simulink model "SPGF_FSK_0000_R2022b"  (R2022b)
settings: Solver=ode4  StartTime=0.0  StopTime=1.4  FixedStep=50e-6/50  RelTol=1e-3  EnableMultiTasking=on
undefined symbols (not defined in the file): D11, Delta
libraries: spsSeriesRLCBranchLib x1646, spsGroundLib x360, spsStairGeneratorLib x147, spsIdealSwitchLib x145, spsCurrentMeasurementLib x145, spsUniversalBridgeLib x76, spsThreePhaseSeriesRLCLoadLib x57, simulink x45, spsBistableLib x36, spsSequenceAnalyzerLib x31, spsThreePhaseParallelRLCLoadLib x20, spsThreePhaseTransformerTwoWindingsLib x20
(part 28 of 40)

== system SPGF_FSK_0000_R2022b/W42/DPL ==
  Ccs2/1 : spsSeriesRLCBranchLib/Series RLC Branch  LConnTagsString=__new0  RConnTagsString=__new0  BranchType=R  Resistance=-Rg_matrix(3,4)*2  Inductance=1e-3  SetiL0=off  InitialCurrent=0  Capacitance=Rg_matrix(3,4)*2  Setx0=off  InitialVoltage=0  Measurements=None
  Ccs2/3 : spsSeriesRLCBranchLib/Series RLC Branch  LConnTagsString=__new0  RConnTagsString=__new0  BranchType=R  Resistance=-Rg_matrix(3,4)*2  Inductance=1e-3  SetiL0=off  InitialCurrent=0  Capacitance=Rg_matrix(3,4)*2  Setx0=off  InitialVoltage=0  Measurements=None
  Ccs3/1 : spsSeriesRLCBranchLib/Series RLC Branch  LConnTagsString=__new0  RConnTagsString=__new0  BranchType=R  Resistance=-Rg_matrix(5,6)*2  Inductance=1e-3  SetiL0=off  InitialCurrent=0  Capacitance=-C_matrix(5,6)/2  Setx0=off  InitialVoltage=0  Measurements=None
  Ccs3/3 : spsSeriesRLCBranchLib/Series RLC Branch  LConnTagsString=__new0  RConnTagsString=__new0  BranchType=R  Resistance=-Rg_matrix(5,6)*2  Inductance=1e-3  SetiL0=off  InitialCurrent=0  Capacitance=-C_matrix(5,6)/2  Setx0=off  InitialVoltage=0  Measurements=None
  DPL : spsDistributedParametersLineLib/Distributed Parameters Line  Phases=6  Length=LineLength  Frequency=Frequency  Resistance=R_matrix  Inductance=L_matrix  Capacitance=C_matrix  x1=[-1.8e-05 -1.53172591975226 5050.73263956514 0 -2664.13868695277 4776.09397012156 0;-1.75e-05 -1.53217240636053 5052.15465053998 0 -2664.88876317377 4775.67515317595 0;-1.7e-05 -1.53261885516397 5053.5765368579 0 -2665.63877364128 4775.25621839527 0;-1.65e-05 -1.53306526615155 5054.99829848381 0 -2666.38871833678 4774.83716578987 0;-1.6e-05 -1.53351163931226 5056.41993538264 0 -2667.13859724178 4774.41799537009 0;-1.55e-05 -1.53395797463509 5057.84144751931 0 -2667.88841033777 4773.99870714626 0;-1.5e-05 -1.53440427210902 5059.26283485875 0 -2668.63815760626 4773.57930112874 0;-1.45e-05 -1.53485053172304 5060.68409736588 0 -2669.38783902873 4773.15977732786 0;-1.4e-05 -1.53529675346615 5062.10523500563 0 -2670.13745458671 4772.74013575399 0;-1.35e-05 -1.53574293732732 5063.52624774295 0 -2670.88700426168 4772.32037641749 0;-1.3e-05 -1.53618908329556 5064.94713554276 0 -2671.63648803516 4771.90049932869 0;-1.25e-05 -1.53663519135985 5066.36789837001 0 -2672.38590588864 4771.48050449797 0;-1.2e-05 -1.53708126150919 5067.78853618965 0 -2673.13525780365 4771.06039193568 0;-1.15e-05 -1.53752729373257 5069.20904896661 0 -2673.8845437617 4770.6401616522 0;-1.1e-05 -1.53797328801899 5070.62943666586 0 -2674.63376374428 4770.2198136579 0;-1.05e-05 -1.53841924435743 5072.04969925233 0 -2675.38291773292 4769.79934796314 0;-1e-05 -1.5388651627369 5073.469836691 0 -2676.13200570914 4769.37876457829 0;-9.5e-06 -1.5393110431464 5074.88984894682 0 -2676.88102765444 4768.95806351374 0;-9e-06 -1.53975688557491 5076.30973598475 0 -2677.62998355035 4768.53724477987 0;-8.5e-06 -1.54020269001145 5077.72949776976 0 -2678.37887337839 4768.11630838706 0;-8e-06 -1.54064845644501 5079.14913426682 0 -2679.12769712009 4767.69525434569 0;-7.5e-06 -1.5410941848646 5080.56864544089 0 -2679.87645475695 4767.27408266616 0;-7e-06 -1.54153987525921 5081.98803125696 0 -2680.62514627051 4766.85279335886 0;-6.5e-06 -1.54198552761784 5083.40729168 0 -2681.3737716423 4766.43138643418 0;-6e-06 -1.54243114192951 5084.82642667499 0 -2682.12233085385 4766.00986190251 0;-5.5e-06 -1.54287671818322 5086.24543620692 0 -2682.87082388668 4765.58821977427 0;-5e-06 -1.54332225636797 5087.66432024077 0 -2683.61925072232 4765.16646005985 0;-4.5e-06 -1.54376775647277 5089.08307874154 0 -2684.36761134231 4764.74458276967 0;-4e-06 -1.54421321848662 5090.50171167422 -12.0892925887177 -2685.11590572819 4764.32258791412 0;-3.5e-06 -1.54465864239855 5091.9202190038 -12.0928204348561 -2685.86413386149 4763.90047550362 0;-3e-06 -1.54510402819755 5093.33860069529 -12.0963479826162 -2686.61229572375 4763.4782455486 0;-2.5e-06 -1.54554937587263 5094.75685671368 -12.0998752319109 -2687.3603912965 4763.05589805946 -9026.79288136857;-2e-06 -1.54599468541281 5096.17498702399 -12.1034021826531 -2688.1084205613 4762.63343304662 -9025.99223903892;-1.5e-06 -1.54643995680711 5097.59299159122 -12.1069288347558 -2688.85638349968 4762.21085052052 -9025.19137400184;-1e-06 -1.54688519004452 5099.01087038039 -12.110455188132 -2689.60428009319 4761.78815049157 -9024.39028627708;-5e-07 -1.54733038511408 5100.4286233565 -12.1139812426947 -2690.35211032337 4761.36533297021 -9023.58897588442]  x2=[-1.8e-05 -1.53125275621797 5053.5845076313 0 -2665.64297802649 4783.13395193963 0;-1.75e-05 -1.53170105381603 5055.00866650009 0 -2666.39418720933 4782.71500217531 0;-1.7e-05 -1.53214931362089 5056.43270064153 0 -2667.14533060154 4782.29593440223 0;-1.65e-05 -1.53259753562148 5057.8566100205 0 -2667.89640818457 4781.87674863072 0;-1.6e-05 -1.53304571980674 5059.28039460186 0 -2668.6474199399 4781.45744487113 0;-1.55e-05 -1.53349386616561 5060.70405435048 0 -2669.39836584899 4781.03802313381 0;-1.5e-05 -1.53394197468704 5062.12758923123 0 -2670.14924589332 4780.61848342911 0;-1.45e-05 -1.53439004535997 5063.55099920899 0 -2670.90006005435 4780.19882576737 0;-1.4e-05 -1.53483807817334 5064.97428424864 0 -2671.65080831357 4779.77905015896 0;-1.35e-05 -1.5352860731161 5066.39744431506 0 -2672.40149065245 4779.35915661423 0;-1.3e-05 -1.53573403017719 5067.82047937313 0 -2673.15210705246 4778.93914514353 0;-1.25e-05 -1.53618194934557 5069.24338938775 0 -2673.90265749509 4778.51901575724 0;-1.2e-05 -1.53662983061017 5070.66617432379 0 -2674.65314196181 4778.09876846572 0;-1.15e-05 -1.53707767395996 5072.08883414617 0 -2675.40356043412 4777.67840327933 0;-1.1e-05 -1.53752547938387 5073.51136881976 0 -2676.15391289349 4777.25792020846 0;-1.05e-05 -1.53797324687086 5074.93377830949 0 -2676.9041993214 4776.83731926347 0;-1e-05 -1.53842097640989 5076.35606258024 0 -2677.65441969936 4776.41660045475 0;-9.5e-06 -1.53886866798989 5077.77822159693 0 -2678.40457400884 4775.99576379267 0;-9e-06 -1.53931632159984 5079.20025532446 0 -2679.15466223133 4775.57480928762 0;-8.5e-06 -1.53976393722868 5080.62216372775 0 -2679.90468434834 4775.15373694998 0;-8e-06 -1.54021151486536 5082.04394677171 0 -2680.65464034134 4774.73254679015 0;-7.5e-06 -1.54065905449885 5083.46560442126 0 -2681.40453019185 4774.31123881852 0;-7e-06 -1.5411065561181 5084.88713664133 0 -2682.15435388134 4773.88981304547 0;-6.5e-06 -1.54155401971207 5086.30854339683 0 -2682.90411139134 4773.46826948142 0;-6e-06 -1.54200144526972 5087.72982465271 0 -2683.65380270333 4773.04660813676 0;-5.5e-06 -1.54244883278001 5089.15098037388 0 -2684.40342779881 4772.6248290219 0;-5e-06 -1.5428961822319 5090.57201052529 0 -2685.1529866593 4772.20293214723 0;-4.5e-06 -1.54334349361435 5091.99291507186 0 -2685.90247926629 4771.78091752318 0;-4e-06 -1.54379076691633 5093.41369397855 -12.0824675797471 -2686.65190560129 4771.35878516016 0;-3.5e-06 -1.5442380021268 5094.83434721029 -12.0860127319719 -2687.40126564582 4770.93653506858 0;-3e-06 -1.54468519923472 5096.25487473204 -12.0895575859862 -2688.15055938137 4770.51416725885 0;-2.5e-06 -1.54513235822907 5097.67527650873 -12.0931021417027 -2688.89978678947 4770.09168174141 -9040.12687605904;-2e-06 -1.5455794790988 5099.09555250533 -12.0966463990338 -2689.64894785163 4769.66907852667 -9039.32597181351;-1.5e-06 -1.54602656183288 5100.51570268679 -12.1001903578921 -2690.39804254936 4769.24635762507 -9038.52484453156;-1e-06 -1.54647360642029 5101.93572701807 -12.1037340181902 -2691.14707086418 4768.82351904703 -9037.72349423295;-5e-07 -1.54692061285 5103.35562546413 -12.1072773798407 -2691.89603277761 4768.40056280298 -9036.92192093744]  x3=[-1.8e-05 0.002122617198667 46.2927341881195 0 -221.66475085935 447.48671858308 0;-1.75e-05 0.00211905638883323 46.3227413419509 0 -221.730346974199 447.449556467 0;-1.7e-05 0.00211549552671385 46.3527473528145 0 -221.79593761807 447.412383310544 0;-1.65e-05 0.00211193461239671 46.3827522199699 0 -221.861522789346 447.37519911463 0;-1.6e-05 0.00210837364596967 46.4127559426767 0 -221.927102486408 447.338003880176 0;-1.55e-05 0.0021048126275206 46.4427585201947 0 -221.992676707639 447.300797608098 0;-1.5e-05 0.00210125155713735 46.4727599517836 0 -222.05824545142 447.263580299316 0;-1.45e-05 0.00209769043490781 46.5027602367031 0 -222.123808716133 447.226351954748 0;-1.4e-05 0.00209412926091982 46.532759374213 0 -222.189366500161 447.189112575312 0;-1.35e-05 0.00209056803526127 46.562757363573 0 -222.254918801887 447.151862161926 0;-1.3e-05 0.00208700675802002 46.5927542040431 0 -222.320465619691 447.114600715511 0;-1.25e-05 0.00208344542928394 46.622749894883 0 -222.386006951959 447.077328236985 0;-1.2e-05 0.0020798840491409 46.6527444353527 0 -222.451542797071 447.040044727268 0;-1.15e-05 0.00207632261767879 46.6827378247121 0 -222.517073153412 447.00275018728 0;-1.1e-05 0.00207276113498546 46.7127300622211 0 -222.582598019364 446.965444617942 0;-1.05e-05 0.00206919960114881 46.7427211471396 0 -222.64811739331 446.928128020173 0;-1e-05 0.0020656380162567 46.7727110787278 0 -222.713631273635 446.890800394894 0;-9.5e-06 0.00206207638039702 46.8026998562456 0 -222.779139658721 446.853461743028 0;-9e-06 0.00205851469365764 46.832687478953 0 -222.844642546952 446.816112065493 0;-8.5e-06 0.00205495295612645 46.8626739461102 0 -222.910139936711 446.778751363214 0;-8e-06 0.00205139116789132 46.8926592569773 0 -222.975631826384 446.74137963711 0;-7.5e-06 0.00204782932904015 46.9226434108144 0 -223.041118214353 446.703996888105 0;-7e-06 0.00204426743966082 46.9526264068816 0 -223.106599099004 446.66660311712 0;-6.5e-06 0.0020407054998412 46.9826082444393 0 -223.17207447872 446.629198325079 0;-6e-06 0.0020371435096692 47.0125889227475 0 -223.237544351885 446.591782512904 0;-5.5e-06 0.0020335814692327 47.0425684410666 0 -223.303008716885 446.554355681519 0;-5e-06 0.00203001937861958 47.0725467986569 0 -223.368467572104 446.516917831846 0;-4.5e-06 0.00202645723791775 47.1025239947787 0 -223.433920915927 446.479468964811 0;-4e-06 0.00202289504721508 47.1325000286922 -0.647291667383035 -223.499368746739 446.442009081335 0;-3.5e-06 0.00201933280659948 47.1624748996579 -0.647579114715986 -223.564811062925 446.404538182345 0;-3e-06 0.00201577051615885 47.1924486069362 -0.647866546070563 -223.630247862871 446.367056268765 0;-2.5e-06 0.00201220817598106 47.2224211497875 -0.648153961439673 -223.695679144961 446.329563341518 -210.051196345615;-2e-06 0.00200864578615404 47.2523925274723 -0.648441360816226 -223.761104907581 446.292059401532 -210.041905260883;-1.5e-06 0.00200508334676566 47.282362739251 -0.648728744193129 -223.826525149118 446.25454444973 -210.032608993574;-1e-06 0.00200152085790383 47.3123317843842 -0.649016111563293 -223.891939867957 446.217018487038 -210.023307543919;-5e-07 0.00199795831965646 47.3422996621324 -0.649303462919625 -223.957349062483 446.179481514383 -210.014000912146]  x4=[-1.8e-05 -0.0220487260336951 80.6197578990134 0 -212.57448045519 393.466897470407 0;-1.75e-05 -0.0220510250408898 80.6255377469379 0 -212.631332867668 393.430432688981 0;-1.7e-05 -0.0220533235039973 80.631315605507 0 -212.688180033678 393.393958200048 0;-1.65e-05 -0.0220556214229608 80.6370914745781 0 -212.745021951818 393.357474004509 0;-1.6e-05 -0.0220579187977237 80.6428653540087 0 -212.801858620684 393.320980103263 0;-1.55e-05 -0.0220602156282293 80.6486372436564 0 -212.858690038876 393.28447649721 0;-1.5e-05 -0.0220625119144208 80.6544071433787 0 -212.915516204989 393.247963187252 0;-1.45e-05 -0.0220648076562417 80.6601750530333 0 -212.972337117623 393.21144017429 0;-1.4e-05 -0.0220671028536353 80.6659409724779 0 -213.029152775375 393.174907459224 0;-1.35e-05 -0.022069397506545 80.6717049015701 0 -213.085963176843 393.138365042956 0;-1.3e-05 -0.0220716916149141 80.6774668401678 0 -213.142768320626 393.101812926388 0;-1.25e-05 -0.022073985178686 80.6832267881288 0 -213.199568205322 393.065251110422 0;-1.2e-05 -0.0220762781978042 80.688984745311 0 -213.25636282953 393.028679595959 0;-1.15e-05 -0.0220785706722121 80.6947407115723 0 -213.313152191847 392.992098383902 0;-1.1e-05 -0.0220808626018531 80.7004946867707 0 -213.369936290874 392.955507475154 0;-1.05e-05 -0.0220831539866706 80.7062466707642 0 -213.426715125208 392.918906870617 0;-1e-05 -0.0220854448266081 80.7119966634109 0 -213.48348869345 392.882296571195 0;-9.5e-06 -0.0220877351216092 80.7177446645689 0 -213.540256994197 392.845676577791 0;-9e-06 -0.0220900248716172 80.7234906740963 0 -213.59702002605 392.809046891309 0;-8.5e-06 -0.0220923140765757 80.7292346918515 0 -213.653777787607 392.772407512651 0;-8e-06 -0.0220946027364282 80.7349767176927 0 -213.710530277469 392.735758442723 0;-7.5e-06 -0.0220968908511182 80.7407167514781 0 -213.767277494235 392.699099682429 0;-7e-06 -0.0220991784205893 80.7464547930662 0 -213.824019436505 392.662431232672 0;-6.5e-06 -0.022101465444785 80.7521908423155 0 -213.880756102879 392.625753094359 0;-6e-06 -0.0221037519236489 80.7579248990843 0 -213.937487491956 392.589065268393 0;-5.5e-06 -0.0221060378571247 80.7636569632311 0 -213.994213602338 392.552367755681 0;-5e-06 -0.0221083232451557 80.7693870346146 0 -214.050934432624 392.515660557127 0;-4.5e-06 -0.0221106080876858 80.7751151130934 0 -214.107649981415 392.478943673637 0;-4e-06 -0.0221128923846585 80.780841198526 -0.795552682406744 -214.164360247311 392.442217106118 0;-3.5e-06 -0.0221151761360175 80.7865652907714 -0.795688042116718 -214.221065228914 392.405480855475 0;-3e-06 -0.0221174593417063 80.7922873896881 -0.795823382193877 -214.277764924823 392.368734922615 0;-2.5e-06 -0.0221197420016687 80.7980074951351 -0.795958702634881 -214.334459333641 392.331979308444 -54.7752950313322;-2e-06 -0.0221220241158484 80.8037256069711 -0.796094003436392 -214.391148453968 392.29521401387 -54.7611320318324;-1.5e-06 -0.022124305684189 80.8094417250551 -0.79622928459507 -214.447832284406 392.2584390398 -54.7469676811557;-1e-06 -0.0221265867066342 80.815155849246 -0.796364546107578 -214.504510823555 392.22165438714 -54.7328019796519;-5e-07 -0.0221288671831278 80.8208679794029 -0.796499787970579 -214.561184070018 392.184860056799 -54.7186349276702]  x5=1.76104117842525e-05  V1=ones(3,3)  V2=ones(3,3)  I1=ones(3,3)  I2=ones(3,3)  nHarmo=1  Measurements=None  Decoupling=off  VsMag0=0  VrMag0=0  VsAngle0=0  VrAngle0=0  IsMag0=0  IrMag0=0  IsAngle0=0  IrAngle0=0
      settings: LibrarySourceBlock=sps_lib/Power Grid Elements/Distributed Parameters Line
  Ground{1..4} (4 alike) : spsGroundLib/Ground  LConnTagsString=a
  Rcs*1 : spsSeriesRLCBranchLib/Series RLC Branch  LConnTagsString=__new0  RConnTagsString=__new0  BranchType=R  Resistance=-Rg_matrix(1,2)*2  Inductance=1e-3  SetiL0=off  InitialCurrent=0  Capacitance=Rg_matrix(1,2)*2  Setx0=off  InitialVoltage=0  Measurements=None
  Rcs*2 : spsSeriesRLCBranchLib/Series RLC Branch  LConnTagsString=__new0  RConnTagsString=__new0  BranchType=R  Resistance=-Rg_matrix(1,2)*2  Inductance=1e-3  SetiL0=off  InitialCurrent=0  Capacitance=Rg_matrix(1,2)*2  Setx0=off  InitialVoltage=0  Measurements=None
  Rgsg1/1 : spsSeriesRLCBranchLib/Series RLC Branch  LConnTagsString=__new0  RConnTagsString=__new0  BranchType=R  Resistance=(Rg_matrix(4,4)+Rg_matrix(3,4))*2  Inductance=1e-3  SetiL0=off  InitialCurrent=0  Capacitance=Rg_matrix(1,2)*2  Setx0=off  InitialVoltage=0  Measurements=None
  Rgsg1/2 : spsSeriesRLCBranchLib/Series RLC Branch  LConnTagsString=__new0  RConnTagsString=__new0  BranchType=R  Resistance=(Rg_matrix(2,2)+Rg_matrix(1,2))*2  Inductance=1e-3  SetiL0=off  InitialCurrent=0  Capacitance=Rg_matrix(1,2)*2  Setx0=off  InitialVoltage=0  Measurements=None
  Rgsg1/3 : spsSeriesRLCBranchLib/Series RLC Branch  LConnTagsString=__new0  RConnTagsString=__new0  BranchType=R  Resistance=(Rg_matrix(4,4)+Rg_matrix(3,4))*2  Inductance=1e-3  SetiL0=off  InitialCurrent=0  Capacitance=Rg_matrix(1,2)*2  Setx0=off  InitialVoltage=0  Measurements=None
  Rgsg1/4 : spsSeriesRLCBranchLib/Series RLC Branch  LConnTagsString=__new0  RConnTagsString=__new0  BranchType=R  Resistance=(Rg_matrix(2,2)+Rg_matrix(1,2))*2  Inductance=1e-3  SetiL0=off  InitialCurrent=0  Capacitance=Rg_matrix(1,2)*2  Setx0=off  InitialVoltage=0  Measurements=None
  Rsg*1 : spsSeriesRLCBranchLib/Series RLC Branch  LConnTagsString=__new0  RConnTagsString=__new0  BranchType=R  Resistance=(Rg_matrix(6,6)+Rg_matrix(5,6))*2  Inductance=1e-3  SetiL0=off  InitialCurrent=0  Capacitance=Rg_matrix(1,2)*2  Setx0=off  InitialVoltage=0  Measurements=None
  Rsg*2 : spsSeriesRLCBranchLib/Series RLC Branch  LConnTagsString=__new0  RConnTagsString=__new0  BranchType=R  Resistance=(Rg_matrix(6,6)+Rg_matrix(5,6))*2  Inductance=1e-3  SetiL0=off  InitialCurrent=0  Capacitance=Rg_matrix(1,2)*2  Setx0=off  InitialVoltage=0  Measurements=None
  A : PMIOPort  Side=Left
  B : PMIOPort  Port=2  Side=Left
  C : PMIOPort  Port=3  Side=Left
  a : PMIOPort  Port=4  Side=Right
  b : PMIOPort  Port=5  Side=Right
  c : PMIOPort  Port=6  Side=Right
  connections:
  c/RConn1 -- Ccs3/1/RConn1 -- DPL/RConn5
  b/RConn1 -- Ccs2/1/RConn1 -- DPL/RConn3
  a/RConn1 -- DPL/RConn1 -- Rcs*1/RConn1
  Ground4/LConn1 -- DPL/RConn6 -- Ccs3/1/LConn1 -- Rsg*1/LConn1 -- Rcs*1/LConn1 -- Rgsg1/4/LConn1 -- DPL/RConn2 -- DPL/RConn4 -- Ccs2/1/LConn1 -- Rgsg1/3/LConn1
  Ground1/LConn1 -- Rgsg1/4/RConn1 -- Rsg*1/RConn1 -- Rgsg1/3/RConn1
  Ground3/LConn1 -- Ccs3/3/LConn1 -- Rsg*2/LConn1 -- DPL/LConn6 -- Rgsg1/1/LConn1 -- Ccs2/3/LConn1 -- DPL/LConn4 -- Rgsg1/2/LConn1 -- Rcs*2/LConn1 -- DPL/LConn2
  Ground2/LConn1 -- Rgsg1/1/RConn1 -- Rsg*2/RConn1 -- Rgsg1/2/RConn1
  Ccs3/3/RConn1 -- DPL/LConn5 -- C/RConn1
  Ccs2/3/RConn1 -- DPL/LConn3 -- B/RConn1
  Rcs*2/RConn1 -- DPL/LConn1 -- A/RConn1

== system SPGF_FSK_0000_R2022b/W42/Pi ==
  Ground{,1..8} (9 alike) : spsGroundLib/Ground  LConnTagsString=a
  Series RLC Branch{,1..2,27..28,33} (6 alike) : spsSeriesRLCBranchLib/Series RLC Branch  LConnTagsString=__new0  RConnTagsString=__new0  BranchType=RL  Resistance=R/2  Inductance=L/2  SetiL0=off  InitialCurrent=0  Capacitance=1e-6  Setx0=off  InitialVoltage=0  Measurements=None
  Series RLC Branch{10..11,13,29..30,32} (6 alike) : spsSeriesRLCBranchLib/Series RLC Branch  LConnTagsString=__new0  RConnTagsString=__new0  BranchType=R  Resistance=Rfg*4  Inductance=L/2  SetiL0=off  InitialCurrent=0  Capacitance=1e-6  Setx0=off  InitialVoltage=0  Measurements=None
  Series RLC Branch{9,12,14,31,40..41} (6 alike) : spsSeriesRLCBranchLib/Series RLC Branch  LConnTagsString=__new0  RConnTagsString=__new0  BranchType=C  Resistance=R/2  Inductance=L/2  SetiL0=off  InitialCurrent=0  Capacitance=Cfg*0.25  Setx0=off  InitialVoltage=0  Measurements=None
  Series RLC Branch15 : spsSeriesRLCBranchLib/Series RLC Branch  LConnTagsString=__new0  RConnTagsString=__new0  BranchType=R  Resistance=Rfg*2  Inductance=L/2  SetiL0=off  InitialCurrent=0  Capacitance=1e-6  Setx0=off  InitialVoltage=0  Measurements=None
  Series RLC Branch16 : spsSeriesRLCBranchLib/Series RLC Branch  LConnTagsString=__new0  RConnTagsString=__new0  BranchType=R  Resistance=Rfg*2  Inductance=L/2  SetiL0=off  InitialCurrent=0  Capacitance=1e-6  Setx0=off  InitialVoltage=0  Measurements=None
  Series RLC Branch17 : spsSeriesRLCBranchLib/Series RLC Branch  LConnTagsString=__new0  RConnTagsString=__new0  BranchType=C  Resistance=R/2  Inductance=L/2  SetiL0=off  InitialCurrent=0  Capacitance=Cfg*0.5  Setx0=off  InitialVoltage=0  Measurements=None
  Series RLC Branch18 : spsSeriesRLCBranchLib/Series RLC Branch  LConnTagsString=__new0  RConnTagsString=__new0  BranchType=R  Resistance=Rfg*2  Inductance=L/2  SetiL0=off  InitialCurrent=0  Capacitance=1e-6  Setx0=off  InitialVoltage=0  Measurements=None
  Series RLC Branch19 : spsSeriesRLCBranchLib/Series RLC Branch  LConnTagsString=__new0  RConnTagsString=__new0  BranchType=C  Resistance=R/2  Inductance=L/2  SetiL0=off  InitialCurrent=0  Capacitance=Cfg*0.5  Setx0=off  InitialVoltage=0  Measurements=None
  Series RLC Branch20 : spsSeriesRLCBranchLib/Series RLC Branch  LConnTagsString=__new0  RConnTagsString=__new0  BranchType=C  Resistance=R/2  Inductance=L/2  SetiL0=off  InitialCurrent=0  Capacitance=Cmf*0.5  Setx0=off  InitialVoltage=0  Measurements=None
  Series RLC Branch21 : spsSeriesRLCBranchLib/Series RLC Branch  LConnTagsString=__new0  RConnTagsString=__new0  BranchType=R  Resistance=Rmf*2  Inductance=L/2  SetiL0=off  InitialCurrent=0  Capacitance=1e-6  Setx0=off  InitialVoltage=0  Measurements=None
  Series RLC Branch22 : spsSeriesRLCBranchLib/Series RLC Branch  LConnTagsString=__new0  RConnTagsString=__new0  BranchType=C  Resistance=R/2  Inductance=L/2  SetiL0=off  InitialCurrent=0  Capacitance=Cmf*0.5  Setx0=off  InitialVoltage=0  Measurements=None
  Series RLC Branch23 : spsSeriesRLCBranchLib/Series RLC Branch  LConnTagsString=__new0  RConnTagsString=__new0  BranchType=R  Resistance=Rmf*2  Inductance=L/2  SetiL0=off  InitialCurrent=0  Capacitance=1e-6  Setx0=off  InitialVoltage=0  Measurements=None
  Series RLC Branch24 : spsSeriesRLCBranchLib/Series RLC Branch  LConnTagsString=__new0  RConnTagsString=__new0  BranchType=C  Resistance=R/2  Inductance=L/2  SetiL0=off  InitialCurrent=0  Capacitance=Cmf*0.5  Setx0=off  InitialVoltage=0  Measurements=None
  Series RLC Branch25 : spsSeriesRLCBranchLib/Series RLC Branch  LConnTagsString=__new0  RConnTagsString=__new0  BranchType=R  Resistance=Rmf*2  Inductance=L/2  SetiL0=off  InitialCurrent=0  Capacitance=1e-6  Setx0=off  InitialVoltage=0  Measurements=None
  Series RLC Branch26 : spsSeriesRLCBranchLib/Series RLC Branch  LConnTagsString=__new0  RConnTagsString=__new0  BranchType=C  Resistance=R/2  Inductance=L/2  SetiL0=off  InitialCurrent=0  Capacitance=Cfg*0.5  Setx0=off  InitialVoltage=0  Measurements=None
  Series RLC Branch{3,5,7,34,36,38} (6 alike) : spsSeriesRLCBranchLib/Series RLC Branch  LConnTagsString=__new0  RConnTagsString=__new0  BranchType=C  Resistance=R/2  Inductance=L/2  SetiL0=off  InitialCurrent=0  Capacitance=Cmf*0.25  Setx0=off  InitialVoltage=0  Measurements=None
  Series RLC Branch{4,6,8,35,37,39} (6 alike) : spsSeriesRLCBranchLib/Series RLC Branch  LConnTagsString=__new0  RConnTagsString=__new0  BranchType=R  Resistance=Rmf*4  Inductance=L/2  SetiL0=off  InitialCurrent=0  Capacitance=1e-6  Setx0=off  InitialVoltage=0  Measurements=None
  A : PMIOPort  Side=Left
  B : PMIOPort  Port=2  Side=Left
  C : PMIOPort  Port=3  Side=Left
  a : PMIOPort  Port=4  Side=Right
  b : PMIOPort  Port=5  Side=Right
  c : PMIOPort  Port=6  Side=Right
  connections:
  Ground8/LConn1 -- Series RLC Branch41/RConn1 -- Series RLC Branch32/RConn1
  Ground7/LConn1 -- Series RLC Branch30/RConn1 -- Series RLC Branch31/RConn1
  Ground6/LConn1 -- Series RLC Branch40/RConn1 -- Series RLC Branch29/RConn1
  Series RLC Branch40/LConn1 -- Series RLC Branch33/RConn1 -- Series RLC Branch38/RConn1 -- Series RLC Branch39/RConn1 -- c/RConn1 -- Series RLC Branch37/RConn1 -- Series RLC Branch36/RConn1 -- Series RLC Branch29/LConn1
  Series RLC Branch35/LConn1 -- Series RLC Branch27/RConn1 -- Series RLC Branch39/LConn1 -- Series RLC Branch38/LConn1 -- Series RLC Branch32/LConn1 -- Series RLC Branch41/LConn1 -- a/RConn1 -- Series RLC Branch34/LConn1
  Series RLC Branch30/LConn1 -- Series RLC Branch28/RConn1 -- Series RLC Branch37/LConn1 -- Series RLC Branch36/LConn1 -- Series RLC Branch34/RConn1 -- Series RLC Branch35/RConn1 -- b/RConn1 -- Series RLC Branch31/LConn1
  Series RLC Branch19/RConn1 -- Series RLC Branch18/RConn1 -- Ground5/LConn1
  Series RLC Branch16/RConn1 -- Series RLC Branch17/RConn1 -- Ground4/LConn1
  Ground3/LConn1 -- Series RLC Branch15/RConn1 -- Series RLC Branch26/RConn1
  Series RLC Branch23/RConn1 -- Series RLC Branch22/RConn1 -- Series RLC Branch24/RConn1 -- Series RLC Branch25/RConn1 -- Series RLC Branch33/LConn1 -- Series RLC Branch2/RConn1 -- Series RLC Branch15/LConn1 -- Series RLC Branch26/LConn1
  Series RLC Branch25/LConn1 -- Series RLC Branch24/LConn1 -- Series RLC Branch18/LConn1 -- Series RLC Branch19/LConn1 -- Series RLC Branch27/LConn1 -- Series RLC Branch/RConn1 -- Series RLC Branch20/LConn1 -- Series RLC Branch21/LConn1
  Series RLC Branch21/RConn1 -- Series RLC Branch20/RConn1 -- Series RLC Branch22/LConn1 -- Series RLC Branch23/LConn1 -- Series RLC Branch1/RConn1 -- Series RLC Branch28/LConn1 -- Series RLC Branch16/LConn1 -- Series RLC Branch17/LConn1
  Ground2/LConn1 -- Series RLC Branch14/RConn1 -- Series RLC Branch13/RConn1
  Ground1/LConn1 -- Series RLC Branch11/RConn1 -- Series RLC Branch12/RConn1
  Series RLC Branch10/RConn1 -- Ground/LConn1 -- Series RLC Branch9/RConn1
  Series RLC Branch10/LConn1 -- Series RLC Branch6/RConn1 -- Series RLC Branch5/RConn1 -- C/RConn1 -- Series RLC Branch7/RConn1 -- Series RLC Branch8/RConn1 -- Series RLC Branch2/LConn1 -- Series RLC Branch9/LConn1
  Series RLC Branch14/LConn1 -- Series RLC Branch/LConn1 -- Series RLC Branch8/LConn1 -- Series RLC Branch7/LConn1 -- Series RLC Branch3/LConn1 -- Series RLC Branch4/LConn1 -- A/RConn1 -- Series RLC Branch13/LConn1
  Series RLC Branch1/LConn1 -- Series RLC Branch3/RConn1 -- Series RLC Branch4/RConn1 -- B/RConn1 -- Series RLC Branch6/LConn1 -- Series RLC Branch5/LConn1 -- Series RLC Branch11/LConn1 -- Series RLC Branch12/LConn1

== system SPGF_FSK_0000_R2022b/W42/Q ==
  breaker : Subsystem  Commented=on  mask{SwitchA=off, SwitchB=off, SwitchC=off, InitialStatus=[1 1 1], BreakerResistance=0.0001, SnubberResistance=1e6, SnubberCapacitance=inf, TransitionTimes=[0.5 0.7], ShiftTimes=[0 0 0]}
      mask prompts: SwitchA "Switching of phase A"; SwitchB "Switching of phase B"; SwitchC "Switching of phase C"; InitialStatus "Initial status of phase breaker [A, B, C]"; BreakerResistance "Breaker resistance Ron (ohms) :"; SnubberResistance "Snubbers resistance Rp (ohms) :"; SnubberCapacitance "Snubbers capacitance Cp (F) :"; TransitionTimes "Transition times (s) :"; ShiftTimes "Time differences for switch [tA, tB, tC] (s) :"
      mask init: same as SPGF_FSK_0000_R2022b/Feed/Q/breaker
      mask Display:
      | % port_label('input',1,'Iabc');
      | 
      | port_label('lconn',1,'A');
      | port_label('lconn',2,'B');
      | port_label('lconn',3,'C');
      | 
      | port_label('rconn',1,'a');
      | port_label('rconn',2,'b');
      | port_label('rconn',3,'c');
      | 
      | disp('   Q    ');
  meas : Subsystem
  shunt : Subsystem
  A : PMIOPort  Side=Right
  B : PMIOPort  Port=2  Side=Right
  C : PMIOPort  Port=3  Side=Right
  a : PMIOPort  Port=4  Side=Left
  b : PMIOPort  Port=5  Side=Left
  c : PMIOPort  Port=6  Side=Left
  connections:
  shunt/LConn3 -- C/RConn1 -- breaker/LConn3
  shunt/LConn2 -- B/RConn1 -- breaker/LConn2
  A/RConn1 -- shunt/LConn1 -- breaker/LConn1
  meas/RConn1 -- a/RConn1
  meas/RConn2 -- b/RConn1
  meas/RConn3 -- c/RConn1
  meas/LConn3 -- breaker/RConn3 -- shunt/RConn3
  meas/LConn2 -- breaker/RConn2 -- shunt/RConn2
  meas/LConn1 -- breaker/RConn1 -- shunt/RConn1

== system SPGF_FSK_0000_R2022b/W42/concentrated ==
  Ccs/1 : spsSeriesRLCBranchLib/Series RLC Branch  LConnTagsString=__new0  RConnTagsString=__new0  BranchType=C  Resistance=190  Inductance=1e-3  SetiL0=off  InitialCurrent=0  Capacitance=-C_matrix(1,2)/2  Setx0=off  InitialVoltage=0  Measurements=None
  Ccs/2 : spsSeriesRLCBranchLib/Series RLC Branch  LConnTagsString=__new0  RConnTagsString=__new0  BranchType=C  Resistance=190  Inductance=1e-3  SetiL0=off  InitialCurrent=0  Capacitance=-C_matrix(1,2)/2  Setx0=off  InitialVoltage=0  Measurements=None
  Ccs2/1 : spsSeriesRLCBranchLib/Series RLC Branch  LConnTagsString=__new0  RConnTagsString=__new0  BranchType=C  Resistance=190  Inductance=1e-3  SetiL0=off  InitialCurrent=0  Capacitance=-C_matrix(3,4)/2  Setx0=off  InitialVoltage=0  Measurements=None
  Ccs2/2 : spsSeriesRLCBranchLib/Series RLC Branch  LConnTagsString=__new0  RConnTagsString=__new0  BranchType=C  Resistance=190  Inductance=1e-3  SetiL0=off  InitialCurrent=0  Capacitance=-C_matrix(3,4)/2  Setx0=off  InitialVoltage=0  Measurements=None
  Ccs2/3 : spsSeriesRLCBranchLib/Series RLC Branch  LConnTagsString=__new0  RConnTagsString=__new0  BranchType=R  Resistance=-Rg_matrix(3,4)*2  Inductance=1e-3  SetiL0=off  InitialCurrent=0  Capacitance=Rg_matrix(3,4)*2  Setx0=off  InitialVoltage=0  Measurements=None
  Ccs2/4 : spsSeriesRLCBranchLib/Series RLC Branch  LConnTagsString=__new0  RConnTagsString=__new0  BranchType=R  Resistance=-Rg_matrix(3,4)*2  Inductance=1e-3  SetiL0=off  InitialCurrent=0  Capacitance=Rg_matrix(3,4)*2  Setx0=off  InitialVoltage=0  Measurements=None
  Ccs3/1 : spsSeriesRLCBranchLib/Series RLC Branch  LConnTagsString=__new0  RConnTagsString=__new0  BranchType=C  Resistance=190  Inductance=1e-3  SetiL0=off  InitialCurrent=0  Capacitance=-C_matrix(5,6)/2  Setx0=off  InitialVoltage=0  Measurements=None
  Ccs3/2 : spsSeriesRLCBranchLib/Series RLC Branch  LConnTagsString=__new0  RConnTagsString=__new0  BranchType=C  Resistance=190  Inductance=1e-3  SetiL0=off  InitialCurrent=0  Capacitance=-C_matrix(5,6)/2  Setx0=off  InitialVoltage=0  Measurements=None
  Ccs3/3 : spsSeriesRLCBranchLib/Series RLC Branch  LConnTagsString=__new0  RConnTagsString=__new0  BranchType=R  Resistance=-Rg_matrix(5,6)*2  Inductance=1e-3  SetiL0=off  InitialCurrent=0  Capacitance=-C_matrix(5,6)/2  Setx0=off  InitialVoltage=0  Measurements=None
  Ccs3/4 : spsSeriesRLCBranchLib/Series RLC Branch  LConnTagsString=__new0  RConnTagsString=__new0  BranchType=R  Resistance=-Rg_matrix(5,6)*2  Inductance=1e-3  SetiL0=off  InitialCurrent=0  Capacitance=-C_matrix(5,6)/2  Setx0=off  InitialVoltage=0  Measurements=None
  Csg/2 : spsSeriesRLCBranchLib/Series RLC Branch  LConnTagsString=__new0  RConnTagsString=__new0  BranchType=C  Resistance=190  Inductance=1e-3  SetiL0=off  InitialCurrent=0  Capacitance=( C_matrix(1,2) + C_matrix(2,2) )/2  Setx0=off  InitialVoltage=0  Measurements=None
  Csg1/1 : spsSeriesRLCBranchLib/Series RLC Branch  LConnTagsString=__new0  RConnTagsString=__new0  BranchType=C  Resistance=190  Inductance=1e-3  SetiL0=off  InitialCurrent=0  Capacitance=( C_matrix(1,2) + C_matrix(2,2) )/2  Setx0=off  InitialVoltage=0  Measurements=None
  Csg2/1 : spsSeriesRLCBranchLib/Series RLC Branch  LConnTagsString=__new0  RConnTagsString=__new0  BranchType=C  Resistance=190  Inductance=1e-3  SetiL0=off  InitialCurrent=0  Capacitance=( C_matrix(3,4) + C_matrix(4,4) )/2  Setx0=off  InitialVoltage=0  Measurements=None
  Csg2/2 : spsSeriesRLCBranchLib/Series RLC Branch  LConnTagsString=__new0  RConnTagsString=__new0  BranchType=C  Resistance=190  Inductance=1e-3  SetiL0=off  InitialCurrent=0  Capacitance=( C_matrix(3,4) + C_matrix(4,4) )/2  Setx0=off  InitialVoltage=0  Measurements=None
  Csg3/1 : spsSeriesRLCBranchLib/Series RLC Branch  LConnTagsString=__new0  RConnTagsString=__new0  BranchType=C  Resistance=190  Inductance=1e-3  SetiL0=off  InitialCurrent=0  Capacitance=( C_matrix(5,6) + C_matrix(6,6) ) /2  Setx0=off  InitialVoltage=0  Measurements=None
  Csg3/2 : spsSeriesRLCBranchLib/Series RLC Branch  LConnTagsString=__new0  RConnTagsString=__new0  BranchType=C  Resistance=190  Inductance=1e-3  SetiL0=off  InitialCurrent=0  Capacitance=( C_matrix(5,6) + C_matrix(6,6) ) /2  Setx0=off  InitialVoltage=0  Measurements=None
  Ground{1..4} (4 alike) : spsGroundLib/Ground  LConnTagsString=a
  RL : spsMutualInductanceLib/Mutual Inductance  LConnTagsString=a|b|c|L4|L5|L6  RConnTagsString=A|B|C|R4|R5|R6  TypeOfMutual=Generalized mutual inductance  NumberOfWindings=6  SelfImpedance1=[1.1 1.1e-03]  SelfImpedance2=[ 1.1 1.1e-03]  ThreeWindings=on  SelfImpedance3=[ 1.1 1.1e-03]  MutualImpedance=[1.0 1.0e-03]  InductanceMatrix=L_matrix  ResistanceMatrix=R_matrix  Measurements=None
      settings: LibrarySourceBlock=sps_lib/Passives/Mutual Inductance
  Rcs*2 : spsSeriesRLCBranchLib/Series RLC Branch  LConnTagsString=__new0  RConnTagsString=__new0  BranchType=R  Resistance=-Rg_matrix(1,2)*2  Inductance=1e-3  SetiL0=off  InitialCurrent=0  Capacitance=Rg_matrix(1,2)*2  Setx0=off  InitialVoltage=0  Measurements=None
  Rgcs1/1 : spsSeriesRLCBranchLib/Series RLC Branch  LConnTagsString=__new0  RConnTagsString=__new0  BranchType=R  Resistance=-Rg_matrix(1,2)*2  Inductance=1e-3  SetiL0=off  InitialCurrent=0  Capacitance=Rg_matrix(1,2)*2  Setx0=off  InitialVoltage=0  Measurements=None
  Rgsg1/1 : spsSeriesRLCBranchLib/Series RLC Branch  LConnTagsString=__new0  RConnTagsString=__new0  BranchType=R  Resistance=(Rg_matrix(4,4)+Rg_matrix(3,4))*2  Inductance=1e-3  SetiL0=off  InitialCurrent=0  Capacitance=Rg_matrix(1,2)*2  Setx0=off  InitialVoltage=0  Measurements=None
  Rgsg1/2 : spsSeriesRLCBranchLib/Series RLC Branch  LConnTagsString=__new0  RConnTagsString=__new0  BranchType=R  Resistance=(Rg_matrix(2,2)+Rg_matrix(1,2))*2  Inductance=1e-3  SetiL0=off  InitialCurrent=0  Capacitance=Rg_matrix(1,2)*2  Setx0=off  InitialVoltage=0  Measurements=None
  Rgsg1/3 : spsSeriesRLCBranchLib/Series RLC Branch  LConnTagsString=__new0  RConnTagsString=__new0  BranchType=R  Resistance=(Rg_matrix(4,4)+Rg_matrix(3,4))*2  Inductance=1e-3  SetiL0=off  InitialCurrent=0  Capacitance=Rg_matrix(1,2)*2  Setx0=off  InitialVoltage=0  Measurements=None
  Rgsg1/4 : spsSeriesRLCBranchLib/Series RLC Branch  LConnTagsString=__new0  RConnTagsString=__new0  BranchType=R  Resistance=(Rg_matrix(2,2)+Rg_matrix(1,2))*2  Inductance=1e-3  SetiL0=off  InitialCurrent=0  Capacitance=Rg_matrix(1,2)*2  Setx0=off  InitialVoltage=0  Measurements=None
  Rsg*2 : spsSeriesRLCBranchLib/Series RLC Branch  LConnTagsString=__new0  RConnTagsString=__new0  BranchType=R  Resistance=(Rg_matrix(6,6)+Rg_matrix(5,6))*2  Inductance=1e-3  SetiL0=off  InitialCurrent=0  Capacitance=Rg_matrix(1,2)*2  Setx0=off  InitialVoltage=0  Measurements=None
  Rsg1/1 : spsSeriesRLCBranchLib/Series RLC Branch  LConnTagsString=__new0  RConnTagsString=__new0  BranchType=R  Resistance=(Rg_matrix(6,6)+Rg_matrix(5,6))*2  Inductance=1e-3  SetiL0=off  InitialCurrent=0  Capacitance=Rg_matrix(1,2)*2  Setx0=off  InitialVoltage=0  Measurements=None
  A : PMIOPort  Side=Left
  B : PMIOPort  Port=2  Side=Left
  C : PMIOPort  Port=3  Side=Left
  a : PMIOPort  Port=4  Side=Right
  b : PMIOPort  Port=5  Side=Right
  c : PMIOPort  Port=6  Side=Right
  connections:
  Ccs3/3/RConn1 -- RL/LConn5 -- C/RConn1 -- Ccs3/2/RConn1
  Ccs2/2/RConn1 -- Ccs2/3/RConn1 -- B/RConn1 -- RL/LConn3
  Ccs/2/RConn1 -- Rcs*2/RConn1 -- A/RConn1 -- RL/LConn1
  Ccs3/4/RConn1 -- RL/RConn5 -- c/RConn1 -- Ccs3/1/RConn1
  Ccs2/1/RConn1 -- Ccs2/4/RConn1 -- RL/RConn3 -- b/RConn1
  Ccs/1/RConn1 -- Rgcs1/1/RConn1 -- RL/RConn1 -- a/RConn1
  Csg/2/RConn1 -- Ground1/LConn1 -- Csg2/2/RConn1 -- Csg3/2/RConn1 -- Rgsg1/2/RConn1 -- Rgsg1/1/RConn1 -- Rsg*2/RConn1
  Csg3/1/LConn1 -- Ccs3/4/LConn1 -- Rsg1/1/LConn1 -- Ccs3/1/LConn1 -- RL/RConn6 -- Ground4/LConn1 -- RL/RConn2 -- Ccs/1/LConn1 -- Csg1/1/LConn1 -- Rgcs1/1/LConn1 -- Rgsg1/4/LConn1 -- RL/RConn4 -- Ccs2/1/LConn1 -- Csg2/1/LConn1 -- Ccs2/4/LConn1 -- Rgsg1/3/LConn1
  Csg1/1/RConn1 -- Ground2/LConn1 -- Csg2/1/RConn1 -- Csg3/1/RConn1 -- Rgsg1/4/RConn1 -- Rgsg1/3/RConn1 -- Rsg1/1/RConn1
  Ccs3/2/LConn1 -- Ccs3/3/LConn1 -- Csg3/2/LConn1 -- Rsg*2/LConn1 -- Ccs2/2/LConn1 -- Ccs2/3/LConn1 -- Csg2/2/LConn1 -- Rgsg1/1/LConn1 -- RL/LConn4 -- RL/LConn2 -- Ccs/2/LConn1 -- Rcs*2/LConn1 -- Csg/2/LConn1 -- Rgsg1/2/LConn1 -- Ground3/LConn1 -- RL/LConn6

== system SPGF_FSK_0000_R2022b/W43/DPL ==
  Ccs2/1 : spsSeriesRLCBranchLib/Series RLC Branch  LConnTagsString=__new0  RConnTagsString=__new0  BranchType=R  Resistance=-Rg_matrix(3,4)*2  Inductance=1e-3  SetiL0=off  InitialCurrent=0  Capacitance=Rg_matrix(3,4)*2  Setx0=off  InitialVoltage=0  Measurements=None
  Ccs2/3 : spsSeriesRLCBranchLib/Series RLC Branch  LConnTagsString=__new0  RConnTagsString=__new0  BranchType=R  Resistance=-Rg_matrix(3,4)*2  Inductance=1e-3  SetiL0=off  InitialCurrent=0  Capacitance=Rg_matrix(3,4)*2  Setx0=off  InitialVoltage=0  Measurements=None
  Ccs3/1 : spsSeriesRLCBranchLib/Series RLC Branch  LConnTagsString=__new0  RConnTagsString=__new0  BranchType=R  Resistance=-Rg_matrix(5,6)*2  Inductance=1e-3  SetiL0=off  InitialCurrent=0  Capacitance=-C_matrix(5,6)/2  Setx0=off  InitialVoltage=0  Measurements=None
  Ccs3/3 : spsSeriesRLCBranchLib/Series RLC Branch  LConnTagsString=__new0  RConnTagsString=__new0  BranchType=R  Resistance=-Rg_matrix(5,6)*2  Inductance=1e-3  SetiL0=off  InitialCurrent=0  Capacitance=-C_matrix(5,6)/2  Setx0=off  InitialVoltage=0  Measurements=None
  DPL : spsDistributedParametersLineLib/Distributed Parameters Line  Phases=6  Length=LineLength  Frequency=Frequency  Resistance=R_matrix  Inductance=L_matrix  Capacitance=C_matrix  x1=[-1.1e-05 -1.53806782779435 0 0 0 0 0;-1.05e-05 -1.53851336069211 0 0 0 0 0;-1e-05 -1.53895885562858 0 0 0 0 0;-9.5e-06 -1.53940431259277 0 0 0 0 0;-9e-06 -1.53984973157367 0 0 0 0 0;-8.5e-06 -1.54029511256031 0 0 0 0 0;-8e-06 -1.54074045554169 0 0 0 0 0;-7.5e-06 -1.54118576050682 0 0 0 0 0;-7e-06 -1.54163102744471 0 0 0 0 0;-6.5e-06 -1.54207625634439 0 0 0 0 0;-6e-06 -1.54252144719486 0 0 0 0 0;-5.5e-06 -1.54296659998513 0 0 0 0 0;-5e-06 -1.54341171470424 0 0 0 0 0;-4.5e-06 -1.54385679134118 0 0 0 0 0;-4e-06 -1.54430182988499 0 0 0 0 0;-3.5e-06 -1.54474683032467 0 0 0 0 0;-3e-06 -1.54519179264926 0 0 0 0 0;-2.5e-06 -1.54563671684776 0 -12.1013617328885 0 0 0;-2e-06 -1.54608160290921 5095.48011910172 -12.1048846370562 -2687.74189462501 4760.98953364988 0;-1.5e-06 -1.54652645082263 5096.89762251466 -12.1084072425479 -2688.48959321668 4760.5669844575 -9022.0759710351;-1e-06 -1.54697126057703 5098.31500016668 -12.1119295492765 -2689.23722547253 4760.14431780284 -9021.27494656023;-5e-07 -1.54741603216145 5099.73225202283 -12.1154515571553 -2689.98479137411 4759.72153369632 -9020.47369949433]  x2=[-1.1e-05 -1.53797328801899 0 0 0 0 0;-1.05e-05 -1.53841924435743 0 0 0 0 0;-1e-05 -1.5388651627369 0 0 0 0 0;-9.5e-06 -1.5393110431464 0 0 0 0 0;-9e-06 -1.53975688557491 0 0 0 0 0;-8.5e-06 -1.54020269001145 0 0 0 0 0;-8e-06 -1.54064845644501 0 0 0 0 0;-7.5e-06 -1.5410941848646 0 0 0 0 0;-7e-06 -1.54153987525921 0 0 0 0 0;-6.5e-06 -1.54198552761784 0 0 0 0 0;-6e-06 -1.54243114192951 0 0 0 0 0;-5.5e-06 -1.54287671818322 0 0 0 0 0;-5e-06 -1.54332225636797 0 0 0 0 0;-4.5e-06 -1.54376775647277 0 0 0 0 0;-4e-06 -1.54421321848662 0 0 0 0 0;-3.5e-06 -1.54465864239855 0 0 0 0 0;-3e-06 -1.54510402819755 0 0 0 0 0;-2.5e-06 -1.54554937587263 0 -12.0998752319109 0 0 0;-2e-06 -1.54599468541281 5096.17498702399 -12.1034021826531 -2688.1084205613 4762.63343304662 0;-1.5e-06 -1.54643995680711 5097.59299159122 -12.1069288347558 -2688.85638349968 4762.21085052052 -9025.19137400184;-1e-06 -1.54688519004452 5099.01087038039 -12.110455188132 -2689.60428009319 4761.78815049157 -9024.39028627708;-5e-07 -1.54733038511408 5100.4286233565 -12.1139812426947 -2690.35211032337 4761.36533297021 -9023.58897588442]  x3=[-1.1e-05 -0.0053314017520819 0 0 0 0 0;-1.05e-05 -0.00533457224199977 0 0 0 0 0;-1e-05 -0.00533774260029235 0 0 0 0 0;-9.5e-06 -0.0053409128268814 0 0 0 0 0;-9e-06 -0.00534408292168871 0 0 0 0 0;-8.5e-06 -0.00534725288463607 0 0 0 0 0;-8e-06 -0.00535042271564524 0 0 0 0 0;-7.5e-06 -0.00535359241463803 0 0 0 0 0;-7e-06 -0.00535676198153622 0 0 0 0 0;-6.5e-06 -0.00535993141626161 0 0 0 0 0;-6e-06 -0.00536310071873599 0 0 0 0 0;-5.5e-06 -0.00536626988888116 0 0 0 0 0;-5e-06 -0.00536943892661893 0 0 0 0 0;-4.5e-06 -0.00537260783187111 0 0 0 0 0;-4e-06 -0.0053757766045595 0 0 0 0 0;-3.5e-06 -0.00537894524460592 0 0 0 0 0;-3e-06 -0.00538211375193219 0 0 0 0 0;-2.5e-06 -0.00538528212646012 0 -0.697342016802859 0 0 0;-2e-06 -0.00538845036811154 57.6439637941706 -0.697583353739372 -222.348611313945 432.361785815105 0;-1.5e-06 -0.00539161847680828 57.666531962225 -0.697824673463705 -222.411703295267 432.324229679048 -162.653915707785;-1e-06 -0.00539478645247217 57.6890987074147 -0.698065975969905 -222.4747897888 432.286662875819 -162.643102505612;-5e-07 -0.00539795429502504 57.7116640291829 -0.698307261252017 -222.537870792988 432.249085406344 -162.632285290381]  x4=[-1.1e-05 -0.0147343083935694 0 0 0 0 0;-1.05e-05 -0.0147369764084132 0 0 0 0 0;-1e-05 -0.0147396440596367 0 0 0 0 0;-9.5e-06 -0.0147423113471741 0 0 0 0 0;-9e-06 -0.0147449782709594 0 0 0 0 0;-8.5e-06 -0.0147476448309271 0 0 0 0 0;-8e-06 -0.0147503110270112 0 0 0 0 0;-7.5e-06 -0.0147529768591459 0 0 0 0 0;-7e-06 -0.0147556423272655 0 0 0 0 0;-6.5e-06 -0.0147583074313043 0 0 0 0 0;-6e-06 -0.0147609721711964 0 0 0 0 0;-5.5e-06 -0.0147636365468762 0 0 0 0 0;-5e-06 -0.0147663005582777 0 0 0 0 0;-4.5e-06 -0.0147689642053355 0 0 0 0 0;-4e-06 -0.0147716274879836 0 0 0 0 0;-3.5e-06 -0.0147742904061565 0 0 0 0 0;-3e-06 -0.0147769529597883 0 0 0 0 0;-2.5e-06 -0.0147796151488135 0 -0.753719575856743 0 0 0;-2e-06 -0.0147822769731663 70.4861182496813 -0.753901300355811 -218.579817156286 411.138304583796 0;-1.5e-06 -0.014784938432781 70.499221110087 -0.754083006253111 -218.639478769549 411.101052699827 -102.048330648584;-1e-06 -0.0147875995275919 70.512322230994 -0.754264693544158 -218.699134988099 411.063790672347 -102.035658323356;-5e-07 -0.0147902602575335 70.5254216120792 -0.754446362224469 -218.758785810463 411.026518502274 -102.0229834805]  x5=1.05662470705515e-05  V1=ones(3,3)  V2=ones(3,3)  I1=ones(3,3)  I2=ones(3,3)  nHarmo=1  Measurements=None  Decoupling=off  VsMag0=0  VrMag0=0  VsAngle0=0  VrAngle0=0  IsMag0=0  IrMag0=0  IsAngle0=0  IrAngle0=0
      settings: LibrarySourceBlock=sps_lib/Power Grid Elements/Distributed Parameters Line
  Ground{1..4} (4 alike) : spsGroundLib/Ground  LConnTagsString=a
  Rcs*1 : spsSeriesRLCBranchLib/Series RLC Branch  LConnTagsString=__new0  RConnTagsString=__new0  BranchType=R  Resistance=-Rg_matrix(1,2)*2  Inductance=1e-3  SetiL0=off  InitialCurrent=0  Capacitance=Rg_matrix(1,2)*2  Setx0=off  InitialVoltage=0  Measurements=None
  Rcs*2 : spsSeriesRLCBranchLib/Series RLC Branch  LConnTagsString=__new0  RConnTagsString=__new0  BranchType=R  Resistance=-Rg_matrix(1,2)*2  Inductance=1e-3  SetiL0=off  InitialCurrent=0  Capacitance=Rg_matrix(1,2)*2  Setx0=off  InitialVoltage=0  Measurements=None
  Rgsg1/1 : spsSeriesRLCBranchLib/Series RLC Branch  LConnTagsString=__new0  RConnTagsString=__new0  BranchType=R  Resistance=(Rg_matrix(4,4)+Rg_matrix(3,4))*2  Inductance=1e-3  SetiL0=off  InitialCurrent=0  Capacitance=Rg_matrix(1,2)*2  Setx0=off  InitialVoltage=0  Measurements=None
  Rgsg1/2 : spsSeriesRLCBranchLib/Series RLC Branch  LConnTagsString=__new0  RConnTagsString=__new0  BranchType=R  Resistance=(Rg_matrix(2,2)+Rg_matrix(1,2))*2  Inductance=1e-3  SetiL0=off  InitialCurrent=0  Capacitance=Rg_matrix(1,2)*2  Setx0=off  InitialVoltage=0  Measurements=None
  Rgsg1/3 : spsSeriesRLCBranchLib/Series RLC Branch  LConnTagsString=__new0  RConnTagsString=__new0  BranchType=R  Resistance=(Rg_matrix(4,4)+Rg_matrix(3,4))*2  Inductance=1e-3  SetiL0=off  InitialCurrent=0  Capacitance=Rg_matrix(1,2)*2  Setx0=off  InitialVoltage=0  Measurements=None
  Rgsg1/4 : spsSeriesRLCBranchLib/Series RLC Branch  LConnTagsString=__new0  RConnTagsString=__new0  BranchType=R  Resistance=(Rg_matrix(2,2)+Rg_matrix(1,2))*2  Inductance=1e-3  SetiL0=off  InitialCurrent=0  Capacitance=Rg_matrix(1,2)*2  Setx0=off  InitialVoltage=0  Measurements=None
  Rsg*1 : spsSeriesRLCBranchLib/Series RLC Branch  LConnTagsString=__new0  RConnTagsString=__new0  BranchType=R  Resistance=(Rg_matrix(6,6)+Rg_matrix(5,6))*2  Inductance=1e-3  SetiL0=off  InitialCurrent=0  Capacitance=Rg_matrix(1,2)*2  Setx0=off  InitialVoltage=0  Measurements=None
  Rsg*2 : spsSeriesRLCBranchLib/Series RLC Branch  LConnTagsString=__new0  RConnTagsString=__new0  BranchType=R  Resistance=(Rg_matrix(6,6)+Rg_matrix(5,6))*2  Inductance=1e-3  SetiL0=off  InitialCurrent=0  Capacitance=Rg_matrix(1,2)*2  Setx0=off  InitialVoltage=0  Measurements=None
  A : PMIOPort  Side=Left
  B : PMIOPort  Port=2  Side=Left
  C : PMIOPort  Port=3  Side=Left
  a : PMIOPort  Port=4  Side=Right
  b : PMIOPort  Port=5  Side=Right
  c : PMIOPort  Port=6  Side=Right
  connections:
  c/RConn1 -- Ccs3/1/RConn1 -- DPL/RConn5
  b/RConn1 -- Ccs2/1/RConn1 -- DPL/RConn3
  a/RConn1 -- DPL/RConn1 -- Rcs*1/RConn1
  Ground4/LConn1 -- DPL/RConn6 -- Ccs3/1/LConn1 -- Rsg*1/LConn1 -- Rcs*1/LConn1 -- Rgsg1/4/LConn1 -- DPL/RConn2 -- DPL/RConn4 -- Ccs2/1/LConn1 -- Rgsg1/3/LConn1
  Ground1/LConn1 -- Rgsg1/4/RConn1 -- Rsg*1/RConn1 -- Rgsg1/3/RConn1
  Ground3/LConn1 -- Ccs3/3/LConn1 -- Rsg*2/LConn1 -- DPL/LConn6 -- Rgsg1/1/LConn1 -- Ccs2/3/LConn1 -- DPL/LConn4 -- Rgsg1/2/LConn1 -- Rcs*2/LConn1 -- DPL/LConn2
  Ground2/LConn1 -- Rgsg1/1/RConn1 -- Rsg*2/RConn1 -- Rgsg1/2/RConn1
  Ccs3/3/RConn1 -- DPL/LConn5 -- C/RConn1
  Ccs2/3/RConn1 -- DPL/LConn3 -- B/RConn1
  Rcs*2/RConn1 -- DPL/LConn1 -- A/RConn1
